simulink model "problem4"  (R2020a)
settings: Solver=VariableStepAuto  StartTime=0.0  StopTime=10.0  RelTol=1e-3
undefined symbols (not defined in the file or in its folder): b, J, K, L, R
settings Model: DataDictionary=datadict.sldd  Creator=Jake  LastModifiedBy=Jake

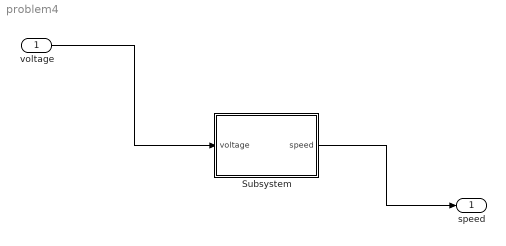
== system problem4 ==
  voltage : Inport
  Subsystem : Subsystem
  speed : Outport
  wires:
  Subsystem/1(speed) -> speed/1
  voltage/1 -> Subsystem/1(voltage)

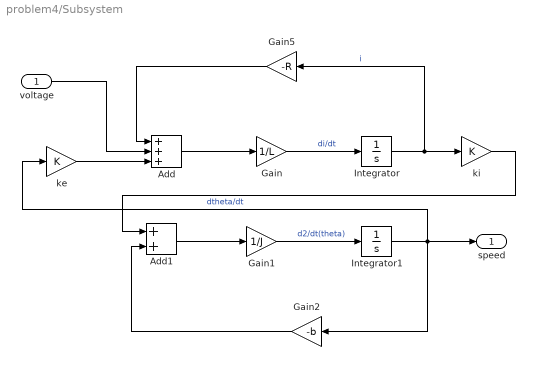
== system problem4/Subsystem ==
  voltage : Inport
  Add : Sum  Inputs=+++
  Add1 : Sum
  Gain : Gain  Gain=1/L
  Gain1 : Gain  Gain=1/J
  Gain2 : Gain  Gain=-b
  Gain5 : Gain  Gain=-R
  Integrator : Integrator
  Integrator1 : Integrator
  ke : Gain  Gain=K
  ki : Gain  Gain=K
  speed : Outport
  wires:
  ke/1 -> Add/3
  Add1/1 -> Gain1/1
  Integrator1/1 -> speed/1, Gain2/1, ke/1  "dtheta/dt"
  Add/1 -> Gain/1
  Integrator/1 -> Gain5/1, ki/1  "i"
  Gain/1 -> Integrator/1  "di/dt"
  Gain1/1 -> Integrator1/1  "d2/dt(theta)"
  Gain2/1 -> Add1/2
  voltage/1 -> Add/2
  ki/1 -> Add1/1
  Gain5/1 -> Add/1
